simulink model "LgV2"  (Simulink 7.3)
settings: Solver=ode3  StartTime=0.0  StopTime=Inf  FixedStep=0.1  RelTol=1e-3
undefined symbols (not defined in the file): eta1_0_real, v1_0_real, velocitySatValues1
libraries: simulink_extras x7, marine_gnc x5, simulink x5, dspinverses x2
(part 2 of 2)

== system LgV2/Plants/CSE1/T_e ==
  -l_x1 : Gain  Gain=-1
  -l_x2 : Gain  Gain=-1
  -l_y2 : Gain  Gain=-1
  3x5 : Reshape  OutputDimensionality=Customize  OutputDimensions=[3,5]
  Mux : Mux  Inputs=15
  T_e{11,13,22,24..25} (5 alike) : Constant
  T_e{12,14..15,21,23} (5 alike) : Constant  Value=0
  l_x1 : Constant  Value=0.425
  l_x2 : Constant  Value=0.425
  l_x3 : Constant  Value=0.425
  l_y1 : Constant  Value=0.055
  l_y2 : Constant  Value=0.055
  T_e : Outport
  wires:
  Mux/1 -> 3x5/1
  3x5/1 -> T_e/1
  T_e11/1 -> Mux/1
  T_e21/1 -> Mux/2
  l_y1/1 -> Mux/3
  T_e12/1 -> Mux/4
  T_e22/1 -> Mux/5
  l_x1/1 -> -l_x1/1
  T_e13/1 -> Mux/7
  T_e23/1 -> Mux/8
  l_y2/1 -> -l_y2/1
  T_e14/1 -> Mux/10
  T_e24/1 -> Mux/11
  l_x2/1 -> -l_x2/1
  T_e15/1 -> Mux/13
  T_e25/1 -> Mux/14
  l_x3/1 -> Mux/15
  -l_x1/1 -> Mux/6
  -l_y2/1 -> Mux/9
  -l_x2/1 -> Mux/12

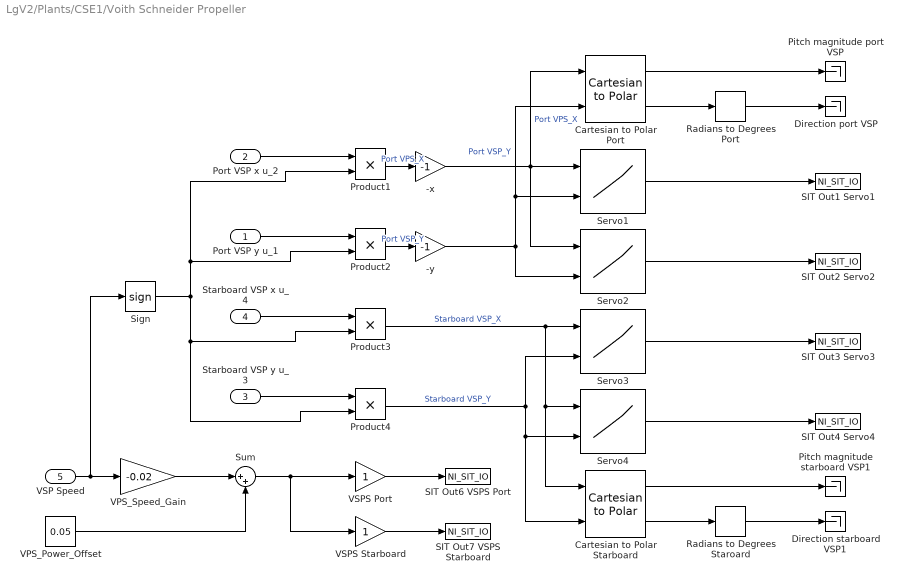
== system LgV2/Plants/CSE1/Voith Schneider Propeller  ==
  Port VSP y u_1 : Inport
  Port VSP x u_2 : Inport  Port=2
  Starboard VSP y u_3 : Inport  Port=3
  Starboard VSP x u_4 : Inport  Port=4
  VSP Speed : Inport  Port=5
  -x : Gain  Gain=-1
  -y : Gain  Gain=-1
  Cartesian to Polar Port : simulink_extras/Transformations/Cartesian to Polar  SystemSampleTime=-1
  Cartesian to Polar Starboard : simulink_extras/Transformations/Cartesian to Polar  SystemSampleTime=-1
  Direction port VSP : Terminator
  Direction starboard VSP1 : Terminator
  Pitch magnitude port VSP : Terminator
  Pitch magnitude starboard VSP1 : Terminator
  Product{1..4} (4 alike) : Product  RndMeth=Zero
  Radians to Degrees Port : simulink_extras/Transformations/Radians to Degrees  SystemSampleTime=-1
  Radians to Degrees Staroard : simulink_extras/Transformations/Radians to Degrees  SystemSampleTime=-1
  SIT Out1 Servo1 : S-Function  Priority=1  FunctionName=NI_SIT_IO  Parameters=width dtype portnum stime stype btype  EnableBusSupport=off  mask(SIT Outport){portnum=1, width=-1, stime=-1, dtype=auto, stype=auto, btype=0}
      mask prompts: portnum "Port number:"; width "Port dimensions (-1 for dynamically sized):"; stime "Sample time (-1 for inherited):"; dtype "Data type:"; stype "Signal type:"; btype "Block type:"
      mask help: Use this outport on any level of nested subsystems to allow the LabVIEW Simulation Interface Toolkit to map hardware to it.
      mask init:
      | NI_SIT_IO_init;
      settings: CopyFcn=NI_SIT_IO_callbacks(1);  DeleteFcn=NI_SIT_IO_callbacks(2);
      mask StyleString: edit,edit,edit,popup(auto|double|single|int8|uint8|int16|uint16|int32|uint32|boolean),popup(auto|real|complex),edit
      mask CallbackString: NI_SIT_IO_callbacks(3);|||NI_SIT_IO_callbacks(4);||
      mask TabNameString: Parameters,Parameters,Parameters,Parameters,Parameters,Parameters
      mask Display:
      | patch([-x x], [-y y], [.90980 .81960 .32156]);
      | plot([0 -x x 0], [rad -y y rad]);
      | fprintf('SIT%d', portnum);
  SIT Out2 Servo2 : S-Function  Priority=2  FunctionName=NI_SIT_IO  Parameters=width dtype portnum stime stype btype  EnableBusSupport=off  mask(SIT Outport){portnum=2, width=-1, stime=-1, dtype=auto, stype=auto, btype=0}
      mask prompts: portnum "Port number:"; width "Port dimensions (-1 for dynamically sized):"; stime "Sample time (-1 for inherited):"; dtype "Data type:"; stype "Signal type:"; btype "Block type:"
      mask help: Use this outport on any level of nested subsystems to allow the LabVIEW Simulation Interface Toolkit to map hardware to it.
      mask init:
      | NI_SIT_IO_init;
      settings: CopyFcn=NI_SIT_IO_callbacks(1);  DeleteFcn=NI_SIT_IO_callbacks(2);
      mask StyleString: edit,edit,edit,popup(auto|double|single|int8|uint8|int16|uint16|int32|uint32|boolean),popup(auto|real|complex),edit
      mask CallbackString: NI_SIT_IO_callbacks(3);|||NI_SIT_IO_callbacks(4);||
      mask TabNameString: Parameters,Parameters,Parameters,Parameters,Parameters,Parameters
      mask Display:
      | patch([-x x], [-y y], [.90980 .81960 .32156]);
      | plot([0 -x x 0], [rad -y y rad]);
      | fprintf('SIT%d', portnum);
  SIT Out3 Servo3 : S-Function  Priority=3  FunctionName=NI_SIT_IO  Parameters=width dtype portnum stime stype btype  EnableBusSupport=off  mask(SIT Outport){portnum=3, width=-1, stime=-1, dtype=auto, stype=auto, btype=0}
      mask prompts: portnum "Port number:"; width "Port dimensions (-1 for dynamically sized):"; stime "Sample time (-1 for inherited):"; dtype "Data type:"; stype "Signal type:"; btype "Block type:"
      mask help: Use this outport on any level of nested subsystems to allow the LabVIEW Simulation Interface Toolkit to map hardware to it.
      mask init:
      | NI_SIT_IO_init;
      settings: CopyFcn=NI_SIT_IO_callbacks(1);  DeleteFcn=NI_SIT_IO_callbacks(2);
      mask StyleString: edit,edit,edit,popup(auto|double|single|int8|uint8|int16|uint16|int32|uint32|boolean),popup(auto|real|complex),edit
      mask CallbackString: NI_SIT_IO_callbacks(3);|||NI_SIT_IO_callbacks(4);||
      mask TabNameString: Parameters,Parameters,Parameters,Parameters,Parameters,Parameters
      mask Display:
      | patch([-x x], [-y y], [.90980 .81960 .32156]);
      | plot([0 -x x 0], [rad -y y rad]);
      | fprintf('SIT%d', portnum);
  SIT Out4 Servo4 : S-Function  Priority=4  FunctionName=NI_SIT_IO  Parameters=width dtype portnum stime stype btype  EnableBusSupport=off  mask(SIT Outport){portnum=4, width=-1, stime=-1, dtype=auto, stype=auto, btype=0}
      mask prompts: portnum "Port number:"; width "Port dimensions (-1 for dynamically sized):"; stime "Sample time (-1 for inherited):"; dtype "Data type:"; stype "Signal type:"; btype "Block type:"
      mask help: Use this outport on any level of nested subsystems to allow the LabVIEW Simulation Interface Toolkit to map hardware to it.
      mask init:
      | NI_SIT_IO_init;
      settings: CopyFcn=NI_SIT_IO_callbacks(1);  DeleteFcn=NI_SIT_IO_callbacks(2);
      mask StyleString: edit,edit,edit,popup(auto|double|single|int8|uint8|int16|uint16|int32|uint32|boolean),popup(auto|real|complex),edit
      mask CallbackString: NI_SIT_IO_callbacks(3);|||NI_SIT_IO_callbacks(4);||
      mask TabNameString: Parameters,Parameters,Parameters,Parameters,Parameters,Parameters
      mask Display:
      | patch([-x x], [-y y], [.90980 .81960 .32156]);
      | plot([0 -x x 0], [rad -y y rad]);
      | fprintf('SIT%d', portnum);
  SIT Out6 VSPS Port : S-Function  Priority=5  FunctionName=NI_SIT_IO  Parameters=width dtype portnum stime stype btype  EnableBusSupport=off  mask(SIT Outport){portnum=5, width=-1, stime=-1, dtype=auto, stype=auto, btype=0}
      mask prompts: portnum "Port number:"; width "Port dimensions (-1 for dynamically sized):"; stime "Sample time (-1 for inherited):"; dtype "Data type:"; stype "Signal type:"; btype "Block type:"
      mask help: Use this outport on any level of nested subsystems to allow the LabVIEW Simulation Interface Toolkit to map hardware to it.
      mask init:
      | NI_SIT_IO_init;
      settings: CopyFcn=NI_SIT_IO_callbacks(1);  DeleteFcn=NI_SIT_IO_callbacks(2);
      mask StyleString: edit,edit,edit,popup(auto|double|single|int8|uint8|int16|uint16|int32|uint32|boolean),popup(auto|real|complex),edit
      mask CallbackString: NI_SIT_IO_callbacks(3);|||NI_SIT_IO_callbacks(4);||
      mask TabNameString: Parameters,Parameters,Parameters,Parameters,Parameters,Parameters
      mask Display:
      | patch([-x x], [-y y], [.90980 .81960 .32156]);
      | plot([0 -x x 0], [rad -y y rad]);
      | fprintf('SIT%d', portnum);
  SIT Out7 VSPS Starboard : S-Function  Priority=6  FunctionName=NI_SIT_IO  Parameters=width dtype portnum stime stype btype  EnableBusSupport=off  mask(SIT Outport){portnum=6, width=-1, stime=-1, dtype=auto, stype=auto, btype=0}
      mask prompts: portnum "Port number:"; width "Port dimensions (-1 for dynamically sized):"; stime "Sample time (-1 for inherited):"; dtype "Data type:"; stype "Signal type:"; btype "Block type:"
      mask help: Use this outport on any level of nested subsystems to allow the LabVIEW Simulation Interface Toolkit to map hardware to it.
      mask init:
      | NI_SIT_IO_init;
      settings: CopyFcn=NI_SIT_IO_callbacks(1);  DeleteFcn=NI_SIT_IO_callbacks(2);
      mask StyleString: edit,edit,edit,popup(auto|double|single|int8|uint8|int16|uint16|int32|uint32|boolean),popup(auto|real|complex),edit
      mask CallbackString: NI_SIT_IO_callbacks(3);|||NI_SIT_IO_callbacks(4);||
      mask TabNameString: Parameters,Parameters,Parameters,Parameters,Parameters,Parameters
      mask Display:
      | patch([-x x], [-y y], [.90980 .81960 .32156]);
      | plot([0 -x x 0], [rad -y y rad]);
      | fprintf('SIT%d', portnum);
  Servo1 : Lookup2D  RowIndex=[-1,0,1]  ColumnIndex=[-1,0,1]  Table=reshape([0.06,0.0495363,0.043301,0.06,0.052446,0.043301,0.06,0.0541518,0.043301],3,3)
  Servo2 : Lookup2D  RowIndex=[-1,0,1]  ColumnIndex=[-1,0,1]  Table=reshape([0.03860880,0.0386088,0.03860880,0.0459941,0.0477243,0.0500953,0.057,0.057,0.057],3,3)
  Servo3 : Lookup2D  RowIndex=[-1,0,1]  ColumnIndex=[-1,0,1]  Table=reshape([0.0640809,0.0640809,0.0640809,0.0539629,0.0541315,0.0556492,0.0442664,0.0442664,0.0442664],3,3)
  Servo4 : Lookup2D  RowIndex=[-1,0,1]  ColumnIndex=[-1,0,1]  Table=reshape([0.0602867,0.0470489,0.0403879,0.0602867,0.049747,0.0403879,0.0602867,0.0526138,0.0403879],3,3)
  Sign : Signum
  Sum : Sum  Inputs=|++
  VPS_Power_Offset : Constant  Value=0.05
  VPS_Speed_Gain : Gain  Gain=-0.02
  VSPS Port : Gain  ParameterDataType=fixdt(1, 16)  ParameterScaling=2^0  OutDataType=fixdt(1, 16)  OutScaling=2^0
  VSPS Starboard : Gain  ParameterDataType=fixdt(1, 16)  ParameterScaling=2^0  OutDataType=fixdt(1, 16)  OutScaling=2^0
  wires:
  Sign/1 -> Product1/2, Product2/2, Product3/2, Product4/2
  Product1/1 -> -x/1  "Port VPS_X"
  Product2/1 -> -y/1  "Port VSP_Y"
  Servo1/1 -> SIT Out1 Servo1/1
  Servo2/1 -> SIT Out2 Servo2/1
  Product3/1 -> Servo3/1, Servo4/1, Cartesian to Polar Starboard/1  "Starboard VSP_X"
  Product4/1 -> Servo3/2, Servo4/2, Cartesian to Polar Starboard/2  "Starboard VSP_Y"
  Servo3/1 -> SIT Out3 Servo3/1
  Servo4/1 -> SIT Out4 Servo4/1
  VSP Speed/1 -> VPS_Speed_Gain/1, Sign/1
  VPS_Speed_Gain/1 -> Sum/1
  VPS_Power_Offset/1 -> Sum/2
  Sum/1 -> VSPS Port/1, VSPS Starboard/1
  -y/1 -> Servo2/2, Servo1/2, Cartesian to Polar Port/2  "Port VSP_Y"
  -x/1 -> Servo1/1, Servo2/1, Cartesian to Polar Port/1  "Port VPS_X"
  Starboard VSP y u_3/1 -> Product4/1
  Starboard VSP x u_4/1 -> Product3/1
  Port VSP y u_1/1 -> Product2/1
  Port VSP x u_2/1 -> Product1/1
  Cartesian to Polar Port/1 -> Pitch magnitude port VSP/1
  Cartesian to Polar Port/2 -> Radians to Degrees Port/1
  Radians to Degrees Port/1 -> Direction port VSP/1
  Cartesian to Polar Starboard/1 -> Pitch magnitude starboard VSP1/1
  Cartesian to Polar Starboard/2 -> Radians to Degrees Staroard/1
  Radians to Degrees Staroard/1 -> Direction starboard VSP1/1
  VSPS Port/1 -> SIT Out6 VSPS Port/1
  VSPS Starboard/1 -> SIT Out7 VSPS Starboard/1

== system LgV2/Plants/Linear Simulator/Vessel Dynamics ==
  tau : Inport
  D_L : Subsystem
  Initial eta : Subsystem
  Initial nu : Subsystem
  Integrator : Integrator  ExternalReset=level  InitialConditionSource=external  InitialCondition=v1_0_real  UpperSaturationLimit=velocitySatValues1  LowerSaturationLimit=-1*velocitySatValues1
  Integrator1 : Integrator  ExternalReset=level  InitialConditionSource=external  InitialCondition=eta1_0_real
  M_inv : Subsystem
  Product1 : Product  Multiplication=Matrix(*)  RndMeth=Zero
  Product2 : Product  Multiplication=Matrix(*)  RndMeth=Zero
  Product3 : Product  Multiplication=Matrix(*)  RndMeth=Zero
  R(psi) : Subsystem
  Reset Linear Simulator integrator : Constant  Value=0
  Sum : Sum  Inputs=+-
  nudot : Terminator
  psi : Selector  InputPortWidth=3  IndexOptions=Index vector (dialog)  Indices=[3]  OutputSizes=1
  eta : Outport
  nu : Outport  Port=2
  etadot : Outport  Port=3
  wires:
  Sum/1 -> Product2/2
  Product2/1 -> Integrator/1, nudot/1
  Integrator/1 -> Product1/2, nu/1, Product3/2
  R(psi)/1(R) -> Product3/1
  psi/1 -> R(psi)/1(psi)
  M_inv/1(M_inv) -> Product2/1
  tau/1 -> Sum/1
  Product1/1 -> Sum/2
  Product3/1 -> etadot/1, Integrator1/1
  Integrator1/1 -> psi/1, eta/1
  Initial nu/1(nu_0) -> Integrator/3
  Reset Linear Simulator integrator/1 -> Integrator/2, Integrator1/2
  Initial eta/1(eta_0) -> Integrator1/3
  D_L/1(D_L) -> Product1/1

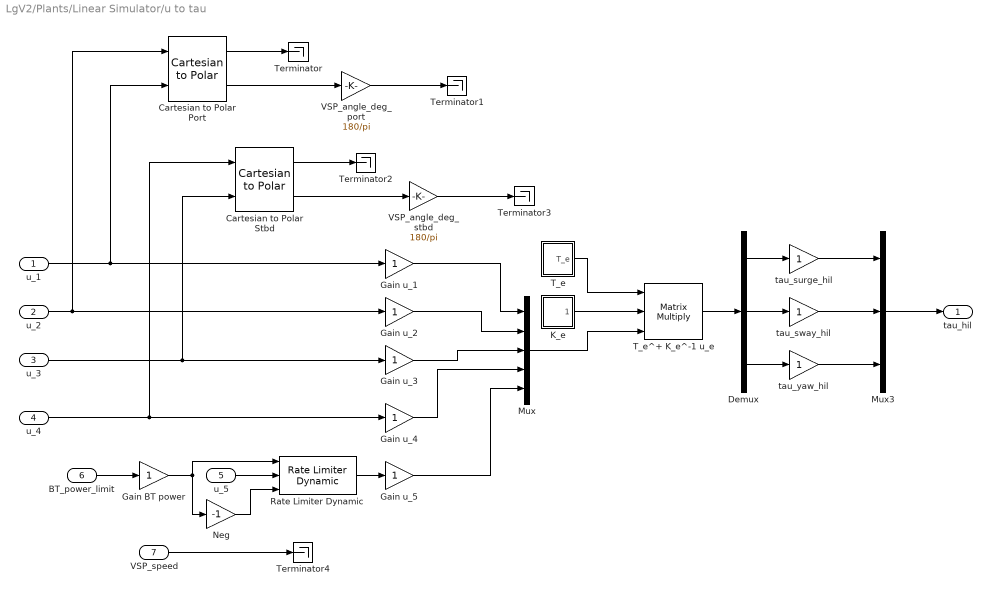
== system LgV2/Plants/Linear Simulator/u to tau ==
  u_1 : Inport
  u_2 : Inport  Port=2
  u_3 : Inport  Port=3
  u_4 : Inport  Port=4
  u_5 : Inport  Port=5
  BT_power_limit : Inport  Port=6
  VSP_speed : Inport  Port=7
  Cartesian to Polar Port : simulink_extras/Transformations/Cartesian to Polar  SystemSampleTime=-1
  Cartesian to Polar Stbd : simulink_extras/Transformations/Cartesian to Polar  SystemSampleTime=-1
  Demux : Demux  Outputs=3
  Gain BT power : Gain  ParameterDataType=fixdt(1, 16)  ParameterScaling=2^0  OutDataType=fixdt(1, 16)  OutScaling=2^0
  Gain u_{1..5} (5 alike) : Gain  ParameterDataType=fixdt(1, 16)  ParameterScaling=2^0  OutDataType=fixdt(1, 16)  OutScaling=2^0
  K_e : Subsystem
  Mux : Mux  Inputs=5
  Mux3 : Mux  Inputs=3
  Neg : Gain  Gain=-1
  Rate Limiter Dynamic : simulink/Discontinuities/Rate Limiter Dynamic  SystemSampleTime=-1
  T_e : Subsystem
  T_e^+ K_e^-1 u_e : Product  Inputs=3  Multiplication=Matrix(*)  RndMeth=Zero
  Terminator{,1..4} (5 alike) : Terminator
  VSP_angle_deg_port : Gain  Gain=180/pi  ParameterDataType=fixdt(1, 16)  ParameterScaling=2^0  OutDataType=fixdt(1, 16)  OutScaling=2^0
  VSP_angle_deg_stbd : Gain  Gain=180/pi  ParameterDataType=fixdt(1, 16)  ParameterScaling=2^0  OutDataType=fixdt(1, 16)  OutScaling=2^0
  tau_surge_hil : Gain  ParameterDataType=fixdt(1, 16)  ParameterScaling=2^0  OutDataType=fixdt(1, 16)  OutScaling=2^0
  tau_sway_hil : Gain  ParameterDataType=fixdt(1, 16)  ParameterScaling=2^0  OutDataType=fixdt(1, 16)  OutScaling=2^0
  tau_yaw_hil : Gain  ParameterDataType=fixdt(1, 16)  ParameterScaling=2^0  OutDataType=fixdt(1, 16)  OutScaling=2^0
  tau_hil : Outport
  wires:
  T_e/1(T_e) -> T_e^+ K_e^-1 u_e/1
  K_e/1(K_e) -> T_e^+ K_e^-1 u_e/2
  VSP_speed/1 -> Terminator4/1
  Neg/1 -> Rate Limiter Dynamic/3
  BT_power_limit/1 -> Gain BT power/1
  u_5/1 -> Rate Limiter Dynamic/2
  Rate Limiter Dynamic/1 -> Gain u_5/1
  Mux/1 -> T_e^+ K_e^-1 u_e/3
  u_1/1 -> Gain u_1/1, Cartesian to Polar Port/2
  u_2/1 -> Gain u_2/1, Cartesian to Polar Port/1
  u_3/1 -> Gain u_3/1, Cartesian to Polar Stbd/2
  u_4/1 -> Gain u_4/1, Cartesian to Polar Stbd/1
  Gain u_1/1 -> Mux/1
  Gain u_2/1 -> Mux/2
  Gain u_3/1 -> Mux/3
  Gain u_4/1 -> Mux/4
  Gain u_5/1 -> Mux/5
  T_e^+ K_e^-1 u_e/1 -> Demux/1
  Demux/1 -> tau_surge_hil/1
  Demux/2 -> tau_sway_hil/1
  Demux/3 -> tau_yaw_hil/1
  tau_surge_hil/1 -> Mux3/1
  tau_sway_hil/1 -> Mux3/2
  tau_yaw_hil/1 -> Mux3/3
  Mux3/1 -> tau_hil/1
  Gain BT power/1 -> Neg/1, Rate Limiter Dynamic/1
  Cartesian to Polar Port/1 -> Terminator/1
  Cartesian to Polar Port/2 -> VSP_angle_deg_port/1
  VSP_angle_deg_port/1 -> Terminator1/1
  Cartesian to Polar Stbd/1 -> Terminator2/1
  Cartesian to Polar Stbd/2 -> VSP_angle_deg_stbd/1
  VSP_angle_deg_stbd/1 -> Terminator3/1

== system LgV2/Plants/Linear Simulator/Vessel Dynamics/D_L ==
  -N_r : Gain  Gain=-1  ParameterDataType=fixdt(1, 16)  ParameterScaling=2^0  OutDataType=fixdt(1, 16)  OutScaling=2^0
  -N_v : Gain  Gain=-1  ParameterDataType=fixdt(1, 16)  ParameterScaling=2^0  OutDataType=fixdt(1, 16)  OutScaling=2^0
  -X_u : Gain  Gain=-1  ParameterDataType=fixdt(1, 16)  ParameterScaling=2^0  OutDataType=fixdt(1, 16)  OutScaling=2^0
  -Y_v : Gain  Gain=-1  ParameterDataType=fixdt(1, 16)  ParameterScaling=2^0  OutDataType=fixdt(1, 16)  OutScaling=2^0
  -Y_vr : Gain  Gain=-1  ParameterDataType=fixdt(1, 16)  ParameterScaling=2^0  OutDataType=fixdt(1, 16)  OutScaling=2^0
  D_L_{12..13,21,31} (4 alike) : Constant  Value=0
  Linear Dampning matrix : Reshape  OutputDimensionality=Customize  OutputDimensions=[3,3]
  Mux : Mux  Inputs=9
  N_r : Constant  Value=-1.900
  N_v : Constant  Value=0.03130
  X_u : Constant  Value=-0.72253
  Y_r : Constant  Value=-7.250
  Y_v : Constant  Value=-0.889656
  D_L : Outport
  wires:
  X_u/1 -> -X_u/1
  Mux/1 -> Linear Dampning matrix/1
  Linear Dampning matrix/1 -> D_L/1
  Y_v/1 -> -Y_v/1
  N_v/1 -> -N_v/1
  Y_r/1 -> -Y_vr/1
  N_r/1 -> -N_r/1
  -X_u/1 -> Mux/1
  D_L_21/1 -> Mux/2
  D_L_31/1 -> Mux/3
  D_L_12/1 -> Mux/4
  -Y_v/1 -> Mux/5
  -N_v/1 -> Mux/6
  D_L_13/1 -> Mux/7
  -Y_vr/1 -> Mux/8
  -N_r/1 -> Mux/9

== system LgV2/Plants/Linear Simulator/Vessel Dynamics/Initial eta ==
  Mux : Mux  Inputs=3
  psi_0 : Constant  Value=0  OutDataType=fixdt(1, 16)  OutScaling=2^0
  x_0 : Constant  Value=0  OutDataType=fixdt(1, 16)  OutScaling=2^0
  y_0 : Constant  Value=0  OutDataType=fixdt(1, 16)  OutScaling=2^0
  eta_0 : Outport  OutDataType=fixdt(1, 16)  OutScaling=2^0
  wires:
  x_0/1 -> Mux/1
  y_0/1 -> Mux/2
  psi_0/1 -> Mux/3
  Mux/1 -> eta_0/1

== system LgV2/Plants/Linear Simulator/Vessel Dynamics/Initial nu ==
  Mux : Mux  Inputs=3
  r_0 : Constant  Value=0  OutDataType=fixdt(1, 16)  OutScaling=2^0
  u_0 : Constant  Value=0  OutDataType=fixdt(1, 16)  OutScaling=2^0
  v_0 : Constant  Value=0  OutDataType=fixdt(1, 16)  OutScaling=2^0
  nu_0 : Outport  OutDataType=fixdt(1, 16)  OutScaling=2^0
  wires:
  u_0/1 -> Mux/1
  v_0/1 -> Mux/2
  r_0/1 -> Mux/3
  Mux/1 -> nu_0/1

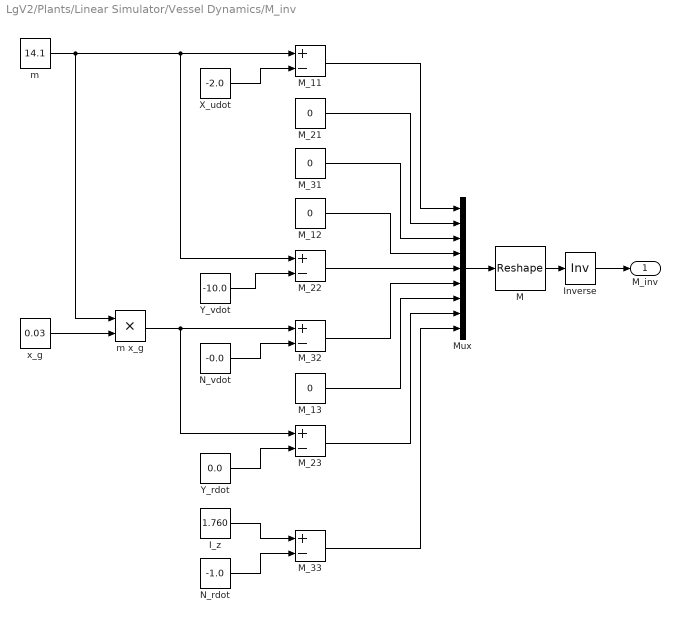
== system LgV2/Plants/Linear Simulator/Vessel Dynamics/M_inv ==
  I_z : Constant  Value=1.760
  Inverse : Product  Inputs=/  Multiplication=Matrix(*)
  M : Reshape  OutputDimensionality=Customize  OutputDimensions=[3,3]
  M_{11,22..23,32..33} (5 alike) : Sum  Inputs=+-
  M_{12..13,21,31} (4 alike) : Constant  Value=0
  Mux : Mux  Inputs=9
  N_rdot : Constant  Value=-1.0
  N_vdot : Constant  Value=-0.0
  X_udot : Constant  Value=-2.0
  Y_rdot : Constant  Value=0.0
  Y_vdot : Constant  Value=-10.0
  m : Constant  Value=14.1
  m x_g : Product  RndMeth=Zero
  x_g : Constant  Value=0.03
  M_inv : Outport
  wires:
  m/1 -> M_11/1, M_22/1, m x_g/1
  X_udot/1 -> M_11/2
  Y_vdot/1 -> M_22/2
  x_g/1 -> m x_g/2
  m x_g/1 -> M_32/1, M_23/1
  N_vdot/1 -> M_32/2
  Y_rdot/1 -> M_23/2
  I_z/1 -> M_33/1
  N_rdot/1 -> M_33/2
  Inverse/1 -> M_inv/1
  M_11/1 -> Mux/1
  M_21/1 -> Mux/2
  M_31/1 -> Mux/3
  M_12/1 -> Mux/4
  M_22/1 -> Mux/5
  M_32/1 -> Mux/6
  M_13/1 -> Mux/7
  M_23/1 -> Mux/8
  M_33/1 -> Mux/9
  Mux/1 -> M/1
  M/1 -> Inverse/1

== system LgV2/Plants/Linear Simulator/Vessel Dynamics/R(psi) ==
  psi : Inport
  Mux : Mux  Inputs=9
  R(psi) : Reshape  OutputDimensionality=Customize  OutputDimensions=[3,3]
  R11 : Fcn  Expr=cos(u(1))
  R12 : Fcn  Expr=-1*sin(u(1))
  R{13,23,31..32} (4 alike) : Constant  Value=0
  R21 : Fcn  Expr=sin(u(1))
  R22 : Fcn  Expr=cos(u(1))
  R33 : Constant
  R : Outport
  wires:
  R(psi)/1 -> R/1
  Mux/1 -> R(psi)/1
  psi/1 -> R11/1, R21/1, R12/1, R22/1
  R11/1 -> Mux/1
  R21/1 -> Mux/2
  R31/1 -> Mux/3
  R12/1 -> Mux/4
  R22/1 -> Mux/5
  R32/1 -> Mux/6
  R13/1 -> Mux/7
  R33/1 -> Mux/9
  R23/1 -> Mux/8

== system LgV2/Plants/Linear Simulator/u to tau/K_e ==
  Constant41 : Constant  Value=0  OutDataType=fixdt(1, 16)  OutScaling=2^0
  Gain K_e1_hil : Gain  ParameterDataType=fixdt(1, 16)  ParameterScaling=2^0  OutDataType=fixdt(1, 16)  OutScaling=2^0
  Gain K_e2_hil : Gain  ParameterDataType=fixdt(1, 16)  ParameterScaling=2^0  OutDataType=fixdt(1, 16)  OutScaling=2^0
  Gain K_e3_hil : Gain  ParameterDataType=fixdt(1, 16)  ParameterScaling=2^0  OutDataType=fixdt(1, 16)  OutScaling=2^0
  Gain K_e4_hil : Gain  ParameterDataType=fixdt(1, 16)  ParameterScaling=2^0  OutDataType=fixdt(1, 16)  OutScaling=2^0
  Gain K_e5_hil : Gain  ParameterDataType=fixdt(1, 16)  ParameterScaling=2^0  OutDataType=fixdt(1, 16)  OutScaling=2^0
  K_e1_hil : Constant  OutDataType=fixdt(1, 16)  OutScaling=2^0
  K_e2_hil : Constant  OutDataType=fixdt(1, 16)  OutScaling=2^0
  K_e3_hil : Constant  OutDataType=fixdt(1, 16)  OutScaling=2^0
  K_e4_hil : Constant  OutDataType=fixdt(1, 16)  OutScaling=2^0
  K_e5_hil : Constant  OutDataType=fixdt(1, 16)  OutScaling=2^0
  Mux12 : Mux  Inputs=25
  Thruster Gain matrix : Reshape  OutputDimensionality=Customize  OutputDimensions=[5,5]
  K_e : Outport  OutDataType=fixdt(1, 16)  OutScaling=2^0
  wires:
  Mux12/1 -> Thruster Gain matrix/1
  K_e1_hil/1 -> Gain K_e1_hil/1
  Thruster Gain matrix/1 -> K_e/1
  Constant41/1 -> Mux12/4, Mux12/2, Mux12/3, Mux12/5, Mux12/6, Mux12/8, Mux12/9, Mux12/10, Mux12/11, Mux12/12, Mux12/14, Mux12/15, Mux12/16, Mux12/17, Mux12/18, Mux12/20, Mux12/21, Mux12/22, Mux12/23, Mux12/24
  K_e2_hil/1 -> Gain K_e2_hil/1
  K_e3_hil/1 -> Gain K_e3_hil/1
  K_e4_hil/1 -> Gain K_e4_hil/1
  K_e5_hil/1 -> Gain K_e5_hil/1
  Gain K_e1_hil/1 -> Mux12/1
  Gain K_e2_hil/1 -> Mux12/7
  Gain K_e3_hil/1 -> Mux12/13
  Gain K_e4_hil/1 -> Mux12/19
  Gain K_e5_hil/1 -> Mux12/25

== system LgV2/Plants/Linear Simulator/u to tau/T_e ==
  -l_x1 : Gain  Gain=-1
  -l_x2 : Gain  Gain=-1
  -l_y2 : Gain  Gain=-1
  3x5 : Reshape  OutputDimensionality=Customize  OutputDimensions=[3,5]
  Mux : Mux  Inputs=15
  T_e{11,13,22,24..25} (5 alike) : Constant
  T_e{12,14..15,21,23} (5 alike) : Constant  Value=0
  l_x1 : Constant  Value=0.425
  l_x2 : Constant  Value=0.425
  l_x3 : Constant  Value=0.425
  l_y1 : Constant  Value=0.055
  l_y2 : Constant  Value=0.055
  T_e : Outport
  wires:
  Mux/1 -> 3x5/1
  3x5/1 -> T_e/1
  T_e11/1 -> Mux/1
  T_e21/1 -> Mux/2
  l_y1/1 -> Mux/3
  T_e12/1 -> Mux/4
  T_e22/1 -> Mux/5
  l_x1/1 -> -l_x1/1
  T_e13/1 -> Mux/7
  T_e23/1 -> Mux/8
  l_y2/1 -> -l_y2/1
  T_e14/1 -> Mux/10
  T_e24/1 -> Mux/11
  l_x2/1 -> -l_x2/1
  T_e15/1 -> Mux/13
  T_e25/1 -> Mux/14
  l_x3/1 -> Mux/15
  -l_x1/1 -> Mux/6
  -l_y2/1 -> Mux/9
  -l_x2/1 -> Mux/12
